simulink model "noCollisionWithRotation"  (R2018a)
settings: Solver=VariableStepAuto  StartTime=0.0  StopTime=inf  RelTol=1e-3
InitFcn:
  | run('initArena.m')
values from neighbouring files (symbols this model uses):
  allObstacles = [1 2 3 4 5 6 7 8 9 10 11 12 ... (3348 elements, 186x3x6)]    [a.mat]    (also in initArena.m = vertcat(limit, obstacle1, obstacle2, obstacle3, obstacle4, o)
  wall = [0 1 2 3 4 5 6 7 8 9 10 11 ... (582 elements, 194x3)]    [a.mat]    (also in initArena.m = generateRectangle(xwall,ywall))
settings Model: Creator=alex  LastModifiedBy=Helen Dekker

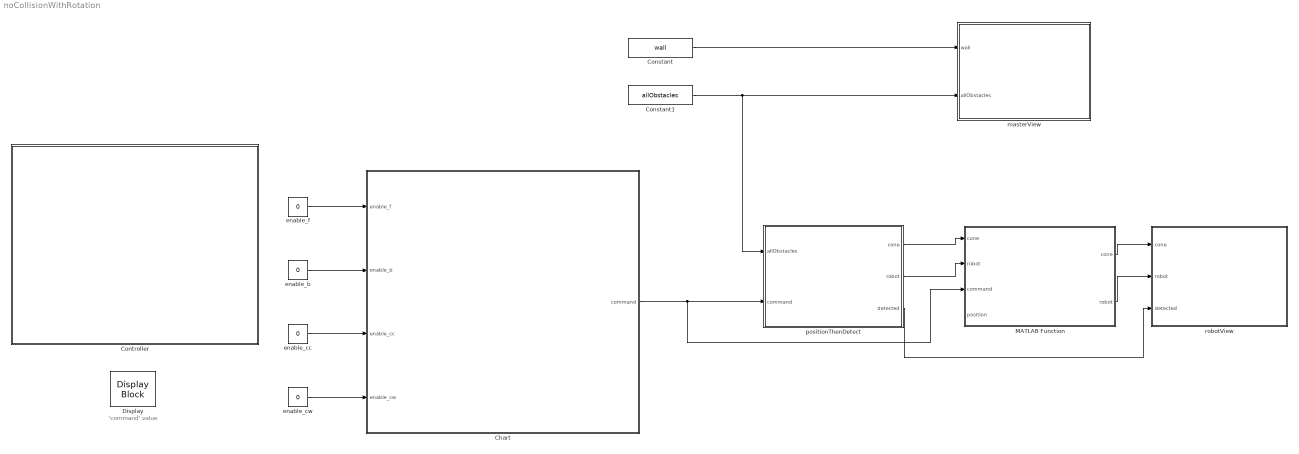
== system noCollisionWithRotation ==
  note: 'command' value
  Chart : Stateflow chart  TreatAsAtomicUnit=on
  Constant : Constant  Value=wall
  Constant1 : Constant  Value=allObstacles
  Controller : Subsystem
  Display : DisplayBlock  WebBlockId=14  LabelPosition=Hide
  MATLAB Function : MATLAB Function  TreatAsAtomicUnit=on
  "enable_b " : Constant  Value=0
  "enable_cc " : Constant  Value=0
  "enable_cw " : Constant  Value=0
  "enable_f " : Constant  Value=0
  masterView : MATLAB Function  TreatAsAtomicUnit=on
  positionThenDetect : MATLAB Function  TreatAsAtomicUnit=on
  robotView : MATLAB Function  TreatAsAtomicUnit=on
  wires:
  "enable_f "/1 -> Chart/1(enable_f)
  "enable_b "/1 -> Chart/2(enable_b)
  "enable_cc "/1 -> Chart/3(enable_cc)
  "enable_cw "/1 -> Chart/4(enable_cw)
  Constant/1 -> masterView/1(wall)
  Constant1/1 -> masterView/2(allObstacles), positionThenDetect/1(allObstacles)
  Chart/1(command) -> MATLAB Function/3(command), positionThenDetect/2(command)
  positionThenDetect/1(cone) -> MATLAB Function/1("cone ")
  positionThenDetect/2(robot) -> MATLAB Function/2("robot ")
  positionThenDetect/3(detected) -> robotView/3(detected)
  MATLAB Function/1(cone) -> robotView/1(cone)
  MATLAB Function/2(robot) -> robotView/2(robot)

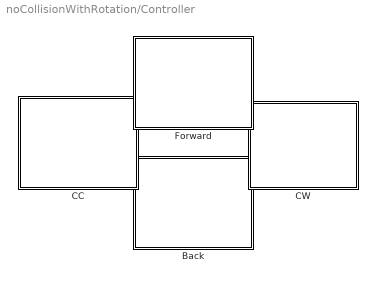
== system noCollisionWithRotation/Controller ==
  Back : Subsystem  DialogController=hmiCreateDDGDialog  IsWebBlock=on  mask(MWDashboardBlock){webBlockId=1a5e94ef-030e-49cd-b944-b929b04abc70, webBlockType=pushbutton, ShowInLibBrwoser=on, ShowInitialText=on, HMISrcModelName=noCollision}
      mask prompts: webBlockId "WebBlock Id"; webBlockType "WebBlock Type"; HMISrcModelName "Source Model"
      mask help: SimulinkHMI:dialogs:PushButtonDialogDesc
      mask Help: helpview([docroot '/mapfiles/simulink.map'], 'hmi_push_button')
      mask Display:
      | model = bdroot(gcb);
      | if strcmp(get_param(model,'BlockDiagramType'), 'library')
      |     image([(matlabroot) '/toolbox/simulink/hmi/icons/PushButton.png']);
      | end
  "CC " : Subsystem  DialogController=hmiCreateDDGDialog  IsWebBlock=on  mask(MWDashboardBlock){webBlockId=f6d6ee6b-2047-45ee-ab2e-570b521bf019, webBlockType=pushbutton, ShowInLibBrwoser=on, ShowInitialText=on, HMISrcModelName=noCollision}
      mask prompts: webBlockId "WebBlock Id"; webBlockType "WebBlock Type"; HMISrcModelName "Source Model"
      mask help: SimulinkHMI:dialogs:PushButtonDialogDesc
      mask Help: helpview([docroot '/mapfiles/simulink.map'], 'hmi_push_button')
      mask Display:
      | model = bdroot(gcb);
      | if strcmp(get_param(model,'BlockDiagramType'), 'library')
      |     image([(matlabroot) '/toolbox/simulink/hmi/icons/PushButton.png']);
      | end
  "CW " : Subsystem  DialogController=hmiCreateDDGDialog  IsWebBlock=on  mask(MWDashboardBlock){webBlockId=5b3cd59d-fae2-469c-adcb-5a1af564bf62, webBlockType=pushbutton, ShowInLibBrwoser=on, ShowInitialText=on, HMISrcModelName=noCollision}
      mask prompts: webBlockId "WebBlock Id"; webBlockType "WebBlock Type"; HMISrcModelName "Source Model"
      mask help: SimulinkHMI:dialogs:PushButtonDialogDesc
      mask Help: helpview([docroot '/mapfiles/simulink.map'], 'hmi_push_button')
      mask Display:
      | model = bdroot(gcb);
      | if strcmp(get_param(model,'BlockDiagramType'), 'library')
      |     image([(matlabroot) '/toolbox/simulink/hmi/icons/PushButton.png']);
      | end
  Forward : Subsystem  DialogController=hmiCreateDDGDialog  IsWebBlock=on  mask(MWDashboardBlock){webBlockId=418d2ee9-92ed-471b-995b-1589f387356b, webBlockType=pushbutton, ShowInLibBrwoser=on, ShowInitialText=on, HMISrcModelName=noCollision}
      mask prompts: webBlockId "WebBlock Id"; webBlockType "WebBlock Type"; HMISrcModelName "Source Model"
      mask help: SimulinkHMI:dialogs:PushButtonDialogDesc
      mask Help: helpview([docroot '/mapfiles/simulink.map'], 'hmi_push_button')
      mask Display:
      | model = bdroot(gcb);
      | if strcmp(get_param(model,'BlockDiagramType'), 'library')
      |     image([(matlabroot) '/toolbox/simulink/hmi/icons/PushButton.png']);
      | end

== system noCollisionWithRotation/Controller/Back ==

== system noCollisionWithRotation/Controller/CC  ==

== system noCollisionWithRotation/Controller/CW  ==

== system noCollisionWithRotation/Controller/Forward ==

== matlab function noCollisionWithRotation/MATLAB Function ==
  data: cone input; cone output; robot input; command input; robot output; position input
function [cone, robot] = rowtayshun (cone, robot, command, position)

tempBot = robot;
tempCone = cone;
if command == 3 % cw
    if position == 1 % "up"
        tempY = tempBot(:,2);
        tempX = tempBot(:,1);
        robot(:,1) = tempY;
        robot(:,2) = tempX;
        
        tempY = tempCone(:,2);
        tempX = tempCone(:,1);
        cone(:,1) = tempY;
        cone(:,2) = tempX;
    elseif position == 2 % "right"
        tempY = tempBot(:,2);
        tempX = tempBot(:,1);
        robot(:,1) = tempY;
        robot(:,2) = tempX*-1;
        
        tempY = tempCone(:,2);
        tempX = tempCone(:,1);
        cone(:,1) = tempY;
        cone(:,2) = tempX*-1;
    elseif position == 3 % "down"
        tempY = tempBot(:,2);
        tempX = tempBot(:,1);
        robot(:,1) = tempY;
        robot(:,2) = tempX;
        
        tempY = tempCone(:,2);
        tempX = tempCone(:,1);
        cone(:,1) = tempY;
        cone(:,2) = tempX;
    elseif position == 4 % "left"
        tempY = tempBot(:,2);
        tempX = tempBot(:,1);
        robot(:,1) = tempY;
        robot(:,2) = tempX*-1;
        
        tempY = tempCone(:,2);
        tempX = tempCone(:,1);
        cone(:,1) = tempY;
        cone(:,2) = tempX*-1;
    end
elseif command == 4 % ccw
    
    if position == 1 % "up"
        tempY = tempBot(:,2);
        tempX = tempBot(:,1);
        robot(:,1) = tempY*-1;
        robot(:,2) = tempX;
        
        tempY = tempCone(:,2);
        tempX = tempCone(:,1);
        cone(:,1) = tempY*-1;
        cone(:,2) = tempX;
    elseif position == 2 % "right"
        tempY = tempBot(:,2);
        tempX = tempBot(:,1);
        robot(:,1) = tempY;
        robot(:,2) = tempX;
        
        tempY = tempCone(:,2);
        tempX = tempCone(:,1);
        cone(:,1) = tempY;
        cone(:,2) = tempX;
    elseif position == 3 % "down"
        tempY = tempBot(:,2);
        tempX = tempBot(:,1);
        robot(:,1) = tempY*-1;
        robot(:,2) = tempX;
        
        tempY = tempCone(:,2);
        tempX = tempCone(:,1);
        cone(:,1) = tempY*-1;
        cone(:,2) = tempX;
    elseif position == 4 % "left"
        tempY = tempBot(:,2);
        tempX = tempBot(:,1);
        robot(:,1) = tempY;
        robot(:,2) = tempX;
        
        tempY = tempCone(:,2);
        tempX = tempCone(:,1);
        cone(:,1) = tempY;
        cone(:,2) = tempX;
    end
end
end

== matlab function noCollisionWithRotation/positionThenDetect ==
  data: allObstacles input; cone output; command input; robot output; detected output
function [cone, robot, detected] = positionThenDetect(allObstacles, command)
    persistent xpos ypos position base_cone base_robot
    
    
    if isempty(xpos)
        xpos = 2000;
        ypos = 2000;
        position = 1;
        % Base vision cone 
        line1 = [0,150,0; 300,450,0;];
        line2 = [0,150,0; -300,450,0;];
        line3 = [-300,450,0; 300,450,0;];
        base_cone = vertcat(line1, line2, line3);

        % Base robot     
        robot_line1 = [0,150,0; 100, 50,0;];
        robot_line2 = [100, 50, 0; 100, -150, 0;];
        robot_line3 = [100, -150, 0; -100, -150, 0;];
        robot_line4 = [-100,-150,0; -100, 50, 0;];
        robot_line5 = [-100, 50, 0; 0, 150, 0;];
        base_robot = vertcat(robot_line1, robot_line2, robot_line3, robot_line4, robot_line5);

    end
    if command ~= 0 
        % Translate base cone and base robot based on x and y positionif command == 1
        % rotate it
        if command == 1 % forwards
            if position == 1 % "up"
                ypos = ypos + 50;
            elseif position == 2 % "right"
                xpos = xpos + 50;
            elseif position == 3 % "down"
                ypos = ypos -50;
            elseif position == 4 % "left"
                xpos = xpos - 50;
            end
        elseif command == 2 % backwards
            if position == 1 % "up"
                ypos = ypos - 50;
            elseif position == 2 % "right"
                xpos = xpos - 50;
            elseif position == 3 % "down"
                ypos = ypos + 50; 
            elseif position == 4 % "left"
                xpos = xpos + 50;
            end
        elseif command == 3 % cw
            [base_cone2, base_robot2] = rowtayshun (base_cone, base_robot, 3, position);
            position = position+1;
            if position == 0
                position = 4;
            end
            if position == 5
                position = 1;
            end
            base_cone = base_cone2;
            base_robot = base_robot2;
        elseif command == 4 % cc
            [base_cone2, base_robot2] = rowtayshun (base_cone, base_robot, 4, position);
            position = position-1; 
            if position == 0
                position = 4;
            end
            if position == 5
                position = 1;
            end
            base_cone = base_cone2;
            base_robot = base_robot2;
        end
    end

    cone = base_cone;
    cone(:,1) = base_cone(:,1) + xpos;
    cone(:,2) = base_cone(:,2) + ypos;
    cone(:,3) = base_cone(:,3);

    robot = base_robot;
    robot(:,1) = base_robot(:,1) + xpos;
    robot(:,2) = base_robot(:,2) + ypos;
    robot(:,3) = base_robot(:,3);

    % Check if obstacle is in vision cone 
    detected = detectObject(allObstacles, cone); 
    
end

== stateflow chart noCollisionWithRotation/Chart ==
  state no_input
    entry: command = 0
  state forward
    entry: command = 1
  state back
    entry: command = 2
  state counter_clockwise
    entry: command = 3
  state clockwise
    entry: command = 3
  (default) -> no_input
  no_input -> forward [order 4] : [enable_f == 1]
  forward -> no_input : [enable_f == 0]
  no_input -> back [order 3] : [enable_b ==1]
  back -> no_input : [enable_b== 0]
  no_input -> counter_clockwise [order 2] : [enable_cc == 1]
  counter_clockwise -> no_input : [enable_cc == 0]
  no_input -> clockwise [order 1] : [enable_cw == 1]
  clockwise -> no_input : [enable_cw == 0]
  data: enable_f input; enable_b input; enable_cc input; enable_cw input; command output

== matlab function noCollisionWithRotation/masterView ==
  data: wall input; allObstacles input
function masterView(wall, allObstacles)
    % Visualize data 
    % hold on
    grid on
    grid minor
    xlim([-800 6600])
    ylim([-700 4400])
    plot(wall(:,1), wall(:,2), 'ks-');
    hold on 
    plot(allObstacles(:,1), allObstacles(:,2), 'bs');
end

== matlab function noCollisionWithRotation/robotView ==
  data: cone input; robot input; detected input
function robotView(cone, robot, detected) 
     if detected
        coneColor = 'r.-';
    else
        coneColor = 'k.-';
    end
    coneFig = plot(cone(:,1), cone(:,2), coneColor); 
    botFig = plot(robot(:,1), robot(:,2), 'k.-');
    set([coneFig botFig],'LineWidth', 5)
    hold off
end
